simulink model "ASM_Traffic_V2X_Complete_Model_2"  (R2019a)
settings: Solver=ode1  StartTime=SIM.tstart.v  StopTime=Inf  FixedStep=SIM.StepSize.v  RelTol=1e-3
PostLoadFcn:
  | if any(exist('dsrtsu_mdlpostloadfcn', 'file') ~= 0), dsrtsu_mdlpostloadfcn('Execute', bdroot); end
  | try, asm_mdl_postloadfcn(bdroot, 'UpdateModel', 2200); catch, disp(lasterr); end,
undefined symbols (not defined in the file): _SensorPnts_1, _SensorPnts_13, _SensorPnts_17, _SensorPnts_21, _SensorPnts_25, _SensorPnts_29, _SensorPnts_33, _SensorPnts_37, _SensorPnts_41, _SensorPnts_45, _SensorPnts_49, _SensorPnts_5, _SensorPnts_53, _SensorPnts_57, _SensorPnts_9, _to_, CPT, G5A, ITS, MDL, rad, s_to_rpm, SIM
libraries: simulink x169, ASM_VehicleDynamics_lib x126, ASM_Traffic_lib x83, ASM_Utils_lib x49, mdbs x45, ASM_Environment_lib x17, dspindex x12, dsaV2xLibraryAux x10, dsmpblib x6, dsaV2xAsn1Library x4, dsaV2xLibrary x4, ASM_BrakeHydraulics_lib x4
(part 13 of 36)

== system ASM_Traffic_V2X_Complete_Model_2/MDL/SoftECU/Soft_ECU_Engine_Basic/StarterPermanentOn_Handling ==
  ASMSignalBus_ : Inport
  Sw_Starter[0Off|1On]_ : Inport  Port=2
  Bus Selector : BusSelector  OutputSignals=Sw_Starter_Mode[1Stim|2PermanentOn]
  BusAssignment : BusAssignment  AssignedSignals=Sw_Starter[0Off|1On]
  StarterPermanantOn : simulink/Logic and Bit Operations/Compare To Constant  relop===  const=2  OutDataTypeStr=boolean
  Sw_StarterOn : Constant
  Switch : Switch  Criteria=u2 ~= 0
  ASMSignalBus : Outport
  Sw_Starter[0Off|1On] : Outport  Port=2
  wires:
  BusAssignment/1 -> ASMSignalBus/1  "EngineOperation"
  Switch/1 -> BusAssignment/2, Sw_Starter[0Off|1On]/1
  Bus Selector/1 -> StarterPermanantOn/1  "<Sw_Starter_Mode[1Stim|2PermanentOn]>"
  Sw_StarterOn/1 -> Switch/1
  StarterPermanantOn/1 -> Switch/2
  ASMSignalBus_/1 -> BusAssignment/1
  [TAG_StartButton_Signals] -> Bus Selector/1
  Sw_Starter[0Off|1On]_/1 -> Switch/3

== system ASM_Traffic_V2X_Complete_Model_2/MDL/SoftECU/Soft_ECU_Engine_Basic/Torque_Intervention_During_Gear_Shift ==
  Factor_Trq_Engine_Red[%] : Inport
  Pos_AccPedal_Driver[%] : Inport  Port=2
  Product : Product
  Saturation[0_100] : Saturate  UpperLimit=100  LowerLimit=0
  UnitConversion : ASM_Utils_lib/UnitConversion/UnitConversion  Selection=%_to_[0_1]
  Pos_AccPedal[%] : Outport
  wires:
  Pos_AccPedal_Driver[%]/1 -> Product/2
  UnitConversion/1 -> Product/1
  Saturation[0_100]/1 -> Pos_AccPedal[%]/1
  Product/1 -> Saturation[0_100]/1
  Factor_Trq_Engine_Red[%]/1 -> UnitConversion/1

== system ASM_Traffic_V2X_Complete_Model_2/MDL/SoftECU/Soft_ECU_Transmission/ASMSignalCollector ==
  BusCreator : BusCreator  Inputs=5
  ASMSignalBus : Outport
  wires:
  BusCreator/1 -> ASMSignalBus/1  "SoftECU_Transmission"
  [ASMBUS_SOFTECU_LOCKUP_CLUTCH_CONTROL] -> BusCreator/1
  [ASMBUS_SOFTECU_SHIFT_LOCK_CONTROL] -> BusCreator/2
  [ASMBUS_SOFTECU_SHIFT_STRATEGY] -> BusCreator/3
  [ASMBUS_SOFTECU_TIP_SHIFT_CONTROL] -> BusCreator/4
  [ASMBUS_SOFTECU_TORQUE_INTERVENTION_CONTROL] -> BusCreator/5

== system ASM_Traffic_V2X_Complete_Model_2/MDL/SoftECU/Soft_ECU_Transmission/SOFTECU_SETUP ==
  Gear_Max_Maneuver[0Off|1_n] : Inport
  SOFTECU_TRANSMISSION_SETUP : ASM_VehicleDynamics_lib/SoftECU/SoftECU_Transmission/SOFTECU_TRANSMISSION_SETUP  Tag=ASM_SUBCOMPONENT  Const_Max_num_Gear=MDL.SoftECU.SoftECUTransmission.Const_Max_num_Gear  ASMProperties=struct('Name','SOFTECU_TRANSMISSION_SETUP','Version','1.0','Library','ASM_VehicleDynamics_lib')  ASMInstanceName=softecu_transmission_setup  ASMInstanceID=1
  Terminator : Terminator
  tag scope: TAG_SoftECU_Const_Max_num_Gear=global
  wires:
  SOFTECU_TRANSMISSION_SETUP/1 -> [TAG_SoftECU_Const_Max_num_Gear]
  [TAG_SoftECU_Const_Max_num_Gear] -> Terminator/1
  Gear_Max_Maneuver[0Off|1_n]/1 -> SOFTECU_TRANSMISSION_SETUP/1

== system ASM_Traffic_V2X_Complete_Model_2/MDL/SoftECU/Soft_ECU_Transmission/Sw_Gear ==
  In[] : Inport
  Ext : Constant
  OR : Logic  Operator=OR  AllPortsSameDT=off  OutDataTypeStr=boolean
  Ref : simulink/Logic and Bit Operations/Compare To Constant  relop===  const=4  OutDataTypeStr=boolean
  SoftECU : Constant  Value=2
  Stim : simulink/Logic and Bit Operations/Compare To Constant  relop===  const=1  OutDataTypeStr=boolean
  Switch : Switch  Criteria=u2 ~= 0
  Terminator : Terminator
  Sw_Gear[] : Outport
  wires:
  Switch/1 -> Terminator/1
  SoftECU/1 -> Switch/3, Sw_Gear[]/1
  Ext/1 -> Switch/1
  OR/1 -> Switch/2
  Ref/1 -> OR/2
  Stim/1 -> OR/1
  In[]/1 -> Ref/1, Stim/1

== system ASM_Traffic_V2X_Complete_Model_2/MDL/SoftECU/Soft_ECU_Transmission/Sw_LockupClutch ==
  In[] : Inport
  SoftECU : Constant  Value=2
  Terminator : Terminator
  Sw_LockupClutch[] : Outport
  wires:
  SoftECU/1 -> Sw_LockupClutch[]/1
  In[]/1 -> Terminator/1

== system ASM_Traffic_V2X_Complete_Model_2/MDL/VehicleDynamics/Brake/ASMSignalCollector ==
  BusCreator3 : BusCreator  Inputs=5
  ASMSignalBus : Outport
  wires:
  BusCreator3/1 -> ASMSignalBus/1  "Brake"
  [ASMBUS_VehicleDynamics_BrakeHydraulics] -> BusCreator3/2
  [TAG_DISP_BrkHyd_MasterBrakeCylinder] -> BusCreator3/1
  [ASMBUS_VehicleDynamics_BrakeDisc] -> BusCreator3/3
  [ASMBUS_VehicleDynamics_BrakeBooster] -> BusCreator3/4
  [ASMBUS_VehicleDynamics_Manifold] -> BusCreator3/5

== system ASM_Traffic_V2X_Complete_Model_2/MDL/VehicleDynamics/Brake/BRAKE_HYDRAULICS ==
  p_MasterBrakeCylinder[bar] : Inport
  Sw_DistributionPattern[1X|2II] : Inport  Port=2
  Reset[] : Inport  Port=3
  Ctrl_HydPump[0_1] : Inport  Port=4
  Ctrl_PreChargeValve_1[] : Inport  Port=5
  Ctrl_PreChargeValve_2[] : Inport  Port=6
  Ctrl_ChangeOverValve_1[] : Inport  Port=7
  Ctrl_ChangeOverValve_2[] : Inport  Port=8
  Ctrl_InletValve_FL[] : Inport  Port=9
  Ctrl_InletValve_FR[] : Inport  Port=10
  Ctrl_InletValve_RL[] : Inport  Port=11
  Ctrl_InletValve_RR[] : Inport  Port=12
  Ctrl_OutletValve_FL[] : Inport  Port=13
  Ctrl_OutletValve_FR[] : Inport  Port=14
  Ctrl_OutletValve_RL[] : Inport  Port=15
  Ctrl_OutletValve_RR[] : Inport  Port=16
  ECU_Mode[0None|1ABS|2ESP|3ASR] : Inport  Port=17
  p_Ambient[bar] : Inport  Port=18
  ASMSignalCollector : Subsystem
  BRAKING_CIRCUIT_BASIC : ASM_BrakeHydraulics_lib/BrakeHydraulics/BrakingCircuitBasic/BRAKING_CIRCUIT_BASIC  Tag=ASM_SUBCOMPONENT  Const_TimeConst=MDL.BrkHyd.BrakeHydraulicsBasic.Const_TimeConst  StepSize=SIM.StepSize  ASMProperties=struct('Name','BRAKING_CIRCUIT_BASIC','Version','4.0','Library','ASM_BrakeHydraulics_lib')  ASMInstanceName=braking_circuit_basic  ASMInstanceID=1
  Mux : Mux
  Mux1 : Mux
  Terminator_{1..2,4,8,11,14} (6 alike) : Terminator
  ASMSignalBus : Outport
  p_Brake[FL,FR,RL,RR][bar] : Outport  Port=2
  tag scope: TAG_DISP_BrkHyd_BrakingCircuitBasic=global
  wires:
  Sw_DistributionPattern[1X|2II]/1 -> Terminator_14/1
  BRAKING_CIRCUIT_BASIC/2 -> p_Brake[FL,FR,RL,RR][bar]/1
  BRAKING_CIRCUIT_BASIC/1 -> [TAG_DISP_BrkHyd_BrakingCircuitBasic]
  Reset[]/1 -> BRAKING_CIRCUIT_BASIC/2
  ASMSignalCollector/1(ASMSignalBus) -> ASMSignalBus/1
  Ctrl_HydPump[0_1]/1 -> Terminator_4/1
  Ctrl_PreChargeValve_1[]/1 -> Terminator_1/1
  Ctrl_ChangeOverValve_1[]/1 -> Terminator_2/1
  Ctrl_PreChargeValve_2[]/1 -> Terminator_11/1
  Ctrl_ChangeOverValve_2[]/1 -> Terminator_8/1
  ECU_Mode[0None|1ABS|2ESP|3ASR]/1 -> BRAKING_CIRCUIT_BASIC/4
  Ctrl_InletValve_FL[]/1 -> Mux/1
  Ctrl_InletValve_FR[]/1 -> Mux/2
  Ctrl_InletValve_RL[]/1 -> Mux/3
  Ctrl_InletValve_RR[]/1 -> Mux/4
  Ctrl_OutletValve_RR[]/1 -> Mux1/4
  Ctrl_OutletValve_RL[]/1 -> Mux1/3
  Ctrl_OutletValve_FR[]/1 -> Mux1/2
  Ctrl_OutletValve_FL[]/1 -> Mux1/1
  Mux/1 -> BRAKING_CIRCUIT_BASIC/5
  Mux1/1 -> BRAKING_CIRCUIT_BASIC/6
  p_Ambient[bar]/1 -> BRAKING_CIRCUIT_BASIC/3
  p_MasterBrakeCylinder[bar]/1 -> BRAKING_CIRCUIT_BASIC/1

== system ASM_Traffic_V2X_Complete_Model_2/MDL/VehicleDynamics/Brake/ForceParkingBrake ==
  Sw_ParkingBrake[0Off|1On] : Inport
  F_ParkingBrake_Off[FL;FR;RL;RR][N] : Constant  Value=[0, 0, 0, 0]
  F_ParkingBrake_On[FL;FR;RL;RR][N] : Constant  Value=[0, 0, 10000, 10000]
  Switch : Switch  Threshold=0.5
  F_ParkingBrake[FL;FR;RL;RR][N] : Outport
  wires:
  Switch/1 -> F_ParkingBrake[FL;FR;RL;RR][N]/1
  F_ParkingBrake_On[FL;FR;RL;RR][N]/1 -> Switch/1
  F_ParkingBrake_Off[FL;FR;RL;RR][N]/1 -> Switch/3
  Sw_ParkingBrake[0Off|1On]/1 -> Switch/2

== system ASM_Traffic_V2X_Complete_Model_2/MDL/VehicleDynamics/Brake/OpenBrkHydModel ==

== system ASM_Traffic_V2X_Complete_Model_2/MDL/VehicleDynamics/CommonVehicleParameters/Rename1 ==
  In1 : Inport
  Out1 : Outport
  wires:
  In1/1 -> Out1/1

== system ASM_Traffic_V2X_Complete_Model_2/MDL/VehicleDynamics/CommonVehicleParameters/Rename2 ==
  In1 : Inport
  Out1 : Outport
  wires:
  In1/1 -> Out1/1

== system ASM_Traffic_V2X_Complete_Model_2/MDL/VehicleDynamics/CommonVehicleParameters/Rename3 ==
  In1 : Inport
  Out1 : Outport
  wires:
  In1/1 -> Out1/1

== system ASM_Traffic_V2X_Complete_Model_2/MDL/VehicleDynamics/CommonVehicleParameters/Rename4 ==
  In1 : Inport
  Out1 : Outport
  wires:
  In1/1 -> Out1/1

== system ASM_Traffic_V2X_Complete_Model_2/MDL/VehicleDynamics/CommonVehicleParameters/Rename5 ==
  In1 : Inport
  Out1 : Outport
  wires:
  In1/1 -> Out1/1

== system ASM_Traffic_V2X_Complete_Model_2/MDL/VehicleDynamics/CommonVehicleParameters/Rename6 ==
  In1 : Inport
  Out1 : Outport
  wires:
  In1/1 -> Out1/1

== system ASM_Traffic_V2X_Complete_Model_2/MDL/VehicleDynamics/CommonVehicleParameters/Rename7 ==
  In1 : Inport
  Out1 : Outport
  wires:
  In1/1 -> Out1/1

== system ASM_Traffic_V2X_Complete_Model_2/MDL/VehicleDynamics/CommonVehicleParameters/Rename8 ==
  In1 : Inport
  Out1 : Outport
  wires:
  In1/1 -> Out1/1

== system ASM_Traffic_V2X_Complete_Model_2/MDL/VehicleDynamics/Suspension/ASMSignalCollector ==
  BusCreator1 : BusCreator  Inputs=2
  ASMSignalBus : Outport
  wires:
  [ASMBUS_SuspensionRear] -> BusCreator1/2
  [ASMBUS_SuspensionFront] -> BusCreator1/1
  BusCreator1/1 -> ASMSignalBus/1  "Suspension"

== system ASM_Traffic_V2X_Complete_Model_2/MDL/VehicleDynamics/Suspension/SuspensionFront ==
  q_Wheel_dt[q1_Front;q2_Front;q1_Rear;q2_Rear][] : Inport
  q_Wheel[q1_Front;q2_Front;q1_Rear;q2_Rear][] : Inport  Port=2
  F_Tire[FL;FR;RL;RR][x;y;z][N] : Inport  Port=3
  Trq_Tire[FL;FR;RL;RR][x;y;z][N|m] : Inport  Port=4
  AirSuspensionSignals_In : Inport  Port=5
  Reset[] : Inport  Port=6
  ASMSignalCollector : Subsystem
  Bus Creator1 : BusCreator  Inputs=8
  Bus Selector4 : BusSelector  OutputSignals=Displ_SteeringRod[Displ;Displ_dt][m;m|s]  OutputAsBus=on
  Constant : Constant  Value=0
  Constant1 : Constant  Value=[0;0]
  Constant2 : Constant  Value=0
  Demux : Demux  Outputs=[1 1]
  Demux1 : Demux  Outputs=[1 1]
  Demux2 : Demux  Outputs=2
  F_FL_dDispl_external[N|m] : Constant  Value=0
  F_FL_external[N] : Constant  Value=0
  F_FR_dDispl_external[N|m] : Constant  Value=0
  F_FR_external[N] : Constant  Value=0
  Mux : Mux  Inputs=2
  Mux1 : Mux  Inputs=2
  Mux2 : Mux  Inputs=2
  OpenSusKinFrontModel : Subsystem
      settings: OpenFcn=asm_open_lib('ASM_VehicleDynamics_lib/VehicleDynamics/Suspension/Front/SuspensionKinematics');
      mask Display: disp('Open\nASM_VehicleDynamics_lib\nSuspension Kinematics Front')
  RELATIVE_POSITION_FRONT : ASM_VehicleDynamics_lib/VehicleDynamics/Suspension/Front/CommonSuspensionBlocks/RELATIVE_POSITION_FRONT  Tag=ASM_SUBCOMPONENT  ASMProperties=struct('Name','RELATIVE_POSITION_FRONT','Version','6.0','Library','ASM_VehicleDynamics_lib')  ASMInstanceName=relative_position_front  ASMInstanceID=1
  RELATIVE_VELOCITIES_FRONT : ASM_VehicleDynamics_lib/VehicleDynamics/Suspension/Front/CommonSuspensionBlocks/RELATIVE_VELOCITIES_FRONT  Tag=ASM_SUBCOMPONENT  ASMProperties=struct('Name','RELATIVE_VELOCITIES_FRONT','Version','3.0','Library','ASM_VehicleDynamics_lib')  ASMInstanceName=relative_velocities_front  ASMInstanceID=1
  STABI_COMP_FRONT : ASM_VehicleDynamics_lib/VehicleDynamics/Suspension/Front/CommonSuspensionBlocks/STABI_COMP_FRONT  ASMProperties=struct('Name','STABI_COMP_FRONT','Version','1.0','Library','ASM_VehicleDynamics_lib')  ASMInstanceName=stabi_comp_front  ASMInstanceID=1
  SUSCOMP_2D_FRONT : ASM_VehicleDynamics_lib/VehicleDynamics/Suspension/Front/CommonSuspensionBlocks/SUSCOMP_2D_FRONT  Tag=ASM_SUBCOMPONENT  Map_Displ_x_Wheel_F_x=MDL.VehicleDynamics.SuspensionCompliance.Front.Map_Displ_x_Wheel_F_x_2d  Map_Displ_x_Wheel_F_y=MDL.VehicleDynamics.SuspensionCompliance.Front.Map_Displ_x_Wheel_F_y_2d  Map_Displ_x_Wheel_Trq_x=MDL.VehicleDynamics.SuspensionCompliance.Front.Map_Displ_x_Wheel_Trq_x_2d  Map_Displ_x_Wheel_Trq_y=MDL.VehicleDynamics.SuspensionCompliance.Front.Map_Displ_x_Wheel_Trq_y_2d  Map_Displ_x_Wheel_Trq_z=MDL.VehicleDynamics.SuspensionCompliance.Front.Map_Displ_x_Wheel_Trq_z_2d  Map_Displ_y_Wheel_F_x=MDL.VehicleDynamics.SuspensionCompliance.Front.Map_Displ_y_Wheel_F_x_2d  Map_Displ_y_Wheel_F_y=MDL.VehicleDynamics.SuspensionCompliance.Front.Map_Displ_y_Wheel_F_y_2d  Map_Displ_y_Wheel_Trq_x=MDL.VehicleDynamics.SuspensionCompliance.Front.Map_Displ_y_Wheel_Trq_x_2d  Map_Displ_y_Wheel_Trq_y=MDL.VehicleDynamics.SuspensionCompliance.Front.Map_Displ_y_Wheel_Trq_y_2d  Map_Displ_y_Wheel_Trq_z=MDL.VehicleDynamics.SuspensionCompliance.Front.Map_Displ_y_Wheel_Trq_z_2d  Map_Angle_Alpha_Wheel_F_x=MDL.VehicleDynamics.SuspensionCompliance.Front.Map_Angle_AlphaCamber_Wheel_F_x_2d  Map_Angle_Alpha_Wheel_F_y=MDL.VehicleDynamics.SuspensionCompliance.Front.Map_Angle_AlphaCamber_Wheel_F_y_2d  Map_Angle_Alpha_Wheel_Trq_x=MDL.VehicleDynamics.SuspensionCompliance.Front.Map_Angle_AlphaCamber_Wheel_Trq_x_2d  Map_Angle_Alpha_Wheel_Trq_y=MDL.VehicleDynamics.SuspensionCompliance.Front.Map_Angle_AlphaCamber_Wheel_Trq_y_2d  Map_Angle_Alpha_Wheel_Trq_z=MDL.VehicleDynamics.SuspensionCompliance.Front.Map_Angle_AlphaCamber_Wheel_Trq_z_2d  Map_Angle_Gamma_Wheel_F_x=MDL.VehicleDynamics.SuspensionCompliance.Front.Map_Angle_GammaToe_Wheel_F_x_2d  Map_Angle_Gamma_Wheel_F_y=MDL.VehicleDynamics.SuspensionCompliance.Front.Map_Angle_GammaToe_Wheel_F_y_2d  Map_Angle_Gamma_Wheel_Trq_x=MDL.VehicleDynamics.SuspensionCompliance.Front.Map_Angle_GammaToe_Wheel_Trq_x_2d  Map_Angle_Gamma_Wheel_Trq_y=MDL.VehicleDynamics.SuspensionCompliance.Front.Map_Angle_GammaToe_Wheel_Trq_y_2d  Map_Angle_Gamma_Wheel_Trq_z=MDL.VehicleDynamics.SuspensionCompliance.Front.Map_Angle_GammaToe_Wheel_Trq_z_2d  Const_NaturalFrequency_Displ_x=MDL.VehicleDynamics.SuspensionCompliance.Front.Const_NaturalFrequency_Displ_x  Const_NaturalFrequency_Displ_y=MDL.VehicleDynamics.SuspensionCompliance.Front.Const_NaturalFrequency_Displ_y  Const_NaturalFrequency_Angle_Alpha=MDL.VehicleDynamics.SuspensionCompliance.Front.Const_NaturalFrequency_Angle_AlphaCamber  Const_NaturalFrequency_Angle_Gamma=MDL.VehicleDynamics.SuspensionCompliance.Front.Const_NaturalFrequency_Angle_GammaToe  StepSize=SIM.StepSize  ASMProperties=struct('Name','SUSCOMP_2D_FRONT','Version','3.0','Library','ASM_VehicleDynamics_lib')  ASMInstanceName=suscomp_2d_front  ASMInstanceID=1
  SUSPENSION_FORCES_FRONT : ASM_VehicleDynamics_lib/VehicleDynamics/Suspension/Front/CommonSuspensionBlocks/SUSPENSION_FORCES_FRONT  Tag=ASM_SUBCOMPONENT  Map_Force_Left_Spring=MDL.VehicleDynamics.Suspension.Front.Map_Force_LeftSpring  Map_Force_Left_Damper=MDL.VehicleDynamics.Suspension.Front.Map_Force_LeftDamper  Map_Force_Right_Spring=MDL.VehicleDynamics.Suspension.Front.Map_Force_RightSpring  Map_Force_Right_Damper=MDL.VehicleDynamics.Suspension.Front.Map_Force_RightDamper  Map_Force_Stabilizer=MDL.VehicleDynamics.Suspension.Front.Map_Force_Stabilizer  ASMProperties=struct('Name','SUSPENSION_FORCES_FRONT','Version','4.0','Library','ASM_VehicleDynamics_lib')  ASMInstanceName=SusForcesFront  ASMInstanceID=1
  SUSPENSION_FORCE_KINEMATICS_FRONT : ASM_VehicleDynamics_lib/VehicleDynamics/Suspension/Front/CommonSuspensionBlocks/SUSPENSION_FORCE_KINEMATICS_FRONT  Tag=ASM_SUBCOMPONENT  StepSize=SIM.StepSize  ASMProperties=struct('Name','SUSPENSION_FORCE_KINEMATICS_FRONT','Version','4.0','Library','ASM_VehicleDynamics_lib')  ASMInstanceName=suspension_force_kinematics_front  ASMInstanceID=1
  SUSPENSION_KINEMATICS_FRONT_SYMMETRIC : ASM_VehicleDynamics_lib/VehicleDynamics/Suspension/Front/SuspensionKinematics/SUSPENSION_KINEMATICS_FRONT_SYMMETRIC  Tag=ASM_SUBCOMPONENT  Const_TrackWidth_Front=MDL.VehicleDynamics.Suspension.Front.TableBased.Const_TrackWidth_Front  Map_Displ_x_Wheel=MDL.VehicleDynamics.Suspension.Front.TableBased.Map_Displ_x_Wheel  Map_Displ_y_Wheel=MDL.VehicleDynamics.Suspension.Front.TableBased.Map_Displ_y_Wheel  Map_Angle_Alpha_Wheel=MDL.VehicleDynamics.Suspension.Front.TableBased.Map_Angle_AlphaCamber_Wheel  Map_Angle_Beta_Wheel=MDL.VehicleDynamics.Suspension.Front.TableBased.Map_Angle_BetaSideView_Wheel  Map_Angle_Gamma_Wheel=MDL.VehicleDynamics.Suspension.Front.TableBased.Map_Angle_GammaToe_Wheel  Map_Displ_Spring=MDL.VehicleDynamics.Suspension.Front.TableBased.Map_Displ_Spring  Map_Displ_Damper=MDL.VehicleDynamics.Suspension.Front.TableBased.Map_Displ_Damper  Map_Displ_Stabilizer=MDL.VehicleDynamics.Suspension.Front.TableBased.Map_Displ_Stabilizer  ASMProperties=struct('Name','SUSPENSION_KINEMATICS_FRONT_SYMMETRIC','Version','10.0','Library','ASM_VehicleDynamics_lib')  ASMInstanceName=SusKinFrontSym  ASMInstanceID=1
  Selector : Selector  InputPortWidth=4  IndexOptions=Index vector (dialog)  Indices=[1 2]  OutputSizes=1
  Selector1 : Selector  InputPortWidth=12  IndexOptions=Index vector (dialog)  Indices=[1 4]  OutputSizes=1
  Selector10 : Selector  InputPortWidth=12  IndexOptions=Index vector (dialog)  Indices=[1 4]  OutputSizes=1
  Selector2 : Selector  InputPortWidth=12  IndexOptions=Index vector (dialog)  Indices=[2 5]  OutputSizes=1
  Selector3 : Selector  InputPortWidth=12  IndexOptions=Index vector (dialog)  Indices=[3 6]  OutputSizes=1
  Selector4 : Selector  InputPortWidth=12  IndexOptions=Index vector (dialog)  Indices=[2 5]  OutputSizes=1
  Selector8 : Selector  InputPortWidth=4  IndexOptions=Index vector (dialog)  Indices=[1 2]  OutputSizes=1
  Sum{,1..3} (4 alike) : Sum  Inputs=++|
  Sum4 : Sum  Inputs=|++
  Terminator : Terminator
  zeros : Constant  Value=zeros(6,1)
  "Pos_Wheel[FL,FR][x;y;z][m] " : Outport
  UnitVec_y_Wheel_CoorSys_V[FL,FR][x;y;z] : Outport  Port=2
  v_Rel_WheelBody[FL,FR][x;y;z][m|s] : Outport  Port=3
  w_Rel_WheelBody[FL,FR][x;y;z][rad|s] : Outport  Port=4
  gF_Front_Susp[q1,q2][] : Outport  Port=5
  gFront_dq_Front_dt[2x2][] : Outport  Port=6
  SuspensionKinematicRelations_Front : Outport  Port=7
  AirSuspensionSignals_Front : Outport  Port=8
  tag scope: ASMBUS_SuspensionComplianceFront=global, ASMBUS_SuspensionForcesFront=global, ASMBUS_SuspensionForcesKinematicsFront=global, ASMBUS_SuspensionKinematicsFront=global, ASMBUS_WheelRelativePositionFront=global, ASMBUS_WheelRelativeVelocityFront=global
  wires:
  Selector4/1 -> SUSCOMP_2D_FRONT/4
  Bus Selector4/1 -> Demux2/1
  [TAG_FromIO_Steering] -> Bus Selector4/1
  STABI_COMP_FRONT/1 -> Sum4/2
  Sum4/1 -> SUSCOMP_2D_FRONT/5
  Selector3/1 -> Sum4/1
  SUSPENSION_KINEMATICS_FRONT_SYMMETRIC/22 -> STABI_COMP_FRONT/1
  Constant2/1 -> AirSuspensionSignals_Front/1
  AirSuspensionSignals_In/1 -> Terminator/1
  Sum3/1 -> SUSPENSION_FORCE_KINEMATICS_FRONT/8
  Sum2/1 -> SUSPENSION_FORCE_KINEMATICS_FRONT/7
  F_FR_dDispl_external[N|m]/1 -> Sum3/1
  F_FR_external[N]/1 -> Sum2/1
  F_FL_dDispl_external[N|m]/1 -> Sum1/1
  Sum1/1 -> SUSPENSION_FORCE_KINEMATICS_FRONT/2
  F_FL_external[N]/1 -> Sum/1
  Sum/1 -> SUSPENSION_FORCE_KINEMATICS_FRONT/1
  Selector10/1 -> SUSCOMP_2D_FRONT/3
  Selector2/1 -> SUSCOMP_2D_FRONT/2
  Selector1/1 -> SUSCOMP_2D_FRONT/1
  Selector8/1 -> Demux1/1
  Selector/1 -> Demux/1
  zeros/1 -> SUSCOMP_2D_FRONT/8
  [TAG_SW_Rotation] -> SUSCOMP_2D_FRONT/7, SUSPENSION_KINEMATICS_FRONT_SYMMETRIC/7, RELATIVE_POSITION_FRONT/9
  Demux2/2 -> Mux2/1, Mux2/2
  Demux2/1 -> Mux/1, Mux/2
  Constant1/1 -> SUSPENSION_FORCE_KINEMATICS_FRONT/21, SUSPENSION_FORCE_KINEMATICS_FRONT/20
  Trq_Tire[FL;FR;RL;RR][x;y;z][N|m]/1 -> Selector3/1, Selector4/1, Selector10/1
  Constant/1 -> SUSPENSION_FORCE_KINEMATICS_FRONT/19, SUSPENSION_FORCE_KINEMATICS_FRONT/18, SUSPENSION_FORCE_KINEMATICS_FRONT/17, SUSPENSION_FORCE_KINEMATICS_FRONT/16
  Reset[]/1 -> SUSCOMP_2D_FRONT/6
  SUSPENSION_FORCE_KINEMATICS_FRONT/2 -> Mux1/1
  SUSPENSION_KINEMATICS_FRONT_SYMMETRIC/1 -> [ASMBUS_SuspensionKinematicsFront]
  SUSPENSION_FORCE_KINEMATICS_FRONT/1 -> [ASMBUS_SuspensionForcesKinematicsFront]
  Demux1/1 -> SUSPENSION_KINEMATICS_FRONT_SYMMETRIC/3
  Demux1/2 -> SUSPENSION_KINEMATICS_FRONT_SYMMETRIC/4
  Demux/1 -> SUSPENSION_KINEMATICS_FRONT_SYMMETRIC/5, RELATIVE_VELOCITIES_FRONT/2
  Demux/2 -> SUSPENSION_KINEMATICS_FRONT_SYMMETRIC/6, RELATIVE_VELOCITIES_FRONT/3
  RELATIVE_VELOCITIES_FRONT/3 -> w_Rel_WheelBody[FL,FR][x;y;z][rad|s]/1
  RELATIVE_VELOCITIES_FRONT/2 -> v_Rel_WheelBody[FL,FR][x;y;z][m|s]/1
  RELATIVE_POSITION_FRONT/1 -> [ASMBUS_WheelRelativePositionFront]
  Bus Creator1/1 -> SuspensionKinematicRelations_Front/1  "SuspensionKinematicRelations_Front"
  SUSPENSION_KINEMATICS_FRONT_SYMMETRIC/9 -> Bus Creator1/8, STABI_COMP_FRONT/3, RELATIVE_VELOCITIES_FRONT/15  "w_Rel_FR_Wheel_dDispl_SteeringRod_dt[x;y;z][rad|m]"
  SUSPENSION_KINEMATICS_FRONT_SYMMETRIC/8 -> RELATIVE_VELOCITIES_FRONT/14, Bus Creator1/7  "w_Rel_FR_Wheel_dq_Front[q1;q2][x;y;z][]"
  SUSPENSION_KINEMATICS_FRONT_SYMMETRIC/7 -> RELATIVE_VELOCITIES_FRONT/13, Bus Creator1/6  "Pos_FR_Wheel_dDispl_SteeringRod[x;y;z][]"
  SUSPENSION_KINEMATICS_FRONT_SYMMETRIC/6 -> RELATIVE_VELOCITIES_FRONT/12, Bus Creator1/5  "Pos_FR_Wheel_dq_Front[q1;q2][x;y;z][]"
  SUSPENSION_KINEMATICS_FRONT_SYMMETRIC/5 -> RELATIVE_VELOCITIES_FRONT/11, Bus Creator1/4, STABI_COMP_FRONT/2  "w_Rel_FL_Wheel_dDispl_SteeringRod_dt[x;y;z][rad|m]"
  SUSPENSION_KINEMATICS_FRONT_SYMMETRIC/4 -> RELATIVE_VELOCITIES_FRONT/10, Bus Creator1/3  "w_Rel_FL_Wheel_dq_Front_dt[q1;q2][x;y;z][]"
  SUSPENSION_KINEMATICS_FRONT_SYMMETRIC/3 -> RELATIVE_VELOCITIES_FRONT/9, Bus Creator1/2  "Pos_FL_Wheel_dDispl_SteeringRod[x;y;z][]"
  SUSPENSION_KINEMATICS_FRONT_SYMMETRIC/2 -> RELATIVE_VELOCITIES_FRONT/8, Bus Creator1/1  "Pos_FL_Wheel_dq_Front[q1;q2][x;y;z][]"
  q_Wheel[q1_Front;q2_Front;q1_Rear;q2_Rear][]/1 -> Selector8/1
  q_Wheel_dt[q1_Front;q2_Front;q1_Rear;q2_Rear][]/1 -> Selector/1
  Mux/1 -> SUSPENSION_KINEMATICS_FRONT_SYMMETRIC/1
  SUSPENSION_FORCE_KINEMATICS_FRONT/4 -> gFront_dq_Front_dt[2x2][]/1
  Mux1/1 -> gF_Front_Susp[q1,q2][]/1
  SUSPENSION_FORCE_KINEMATICS_FRONT/3 -> Mux1/2
  RELATIVE_POSITION_FRONT/3 -> UnitVec_y_Wheel_CoorSys_V[FL,FR][x;y;z]/1
  RELATIVE_POSITION_FRONT/2 -> "Pos_Wheel[FL,FR][x;y;z][m] "/1
  SUSPENSION_KINEMATICS_FRONT_SYMMETRIC/21 -> SUSPENSION_FORCE_KINEMATICS_FRONT/15
  SUSPENSION_KINEMATICS_FRONT_SYMMETRIC/20 -> SUSPENSION_FORCE_KINEMATICS_FRONT/14
  SUSPENSION_KINEMATICS_FRONT_SYMMETRIC/19 -> SUSPENSION_FORCE_KINEMATICS_FRONT/13
  SUSPENSION_KINEMATICS_FRONT_SYMMETRIC/18 -> SUSPENSION_FORCE_KINEMATICS_FRONT/12
  SUSPENSION_KINEMATICS_FRONT_SYMMETRIC/17 -> SUSPENSION_FORCE_KINEMATICS_FRONT/11
  SUSPENSION_FORCES_FRONT/11 -> SUSPENSION_FORCE_KINEMATICS_FRONT/10
  SUSPENSION_FORCES_FRONT/10 -> SUSPENSION_FORCE_KINEMATICS_FRONT/9
  SUSPENSION_FORCES_FRONT/9 -> Sum3/2
  SUSPENSION_FORCES_FRONT/8 -> Sum2/2
  SUSPENSION_FORCES_FRONT/7 -> SUSPENSION_FORCE_KINEMATICS_FRONT/6
  SUSPENSION_FORCES_FRONT/6 -> SUSPENSION_FORCE_KINEMATICS_FRONT/5, STABI_COMP_FRONT/4
  SUSPENSION_FORCES_FRONT/5 -> SUSPENSION_FORCE_KINEMATICS_FRONT/4
  SUSPENSION_FORCES_FRONT/4 -> SUSPENSION_FORCE_KINEMATICS_FRONT/3
  SUSPENSION_FORCES_FRONT/3 -> Sum1/2
  SUSPENSION_FORCES_FRONT/2 -> Sum/2
  SUSPENSION_KINEMATICS_FRONT_SYMMETRIC/16 -> SUSPENSION_FORCES_FRONT/3
  SUSPENSION_KINEMATICS_FRONT_SYMMETRIC/15 -> SUSPENSION_FORCES_FRONT/2
  SUSPENSION_KINEMATICS_FRONT_SYMMETRIC/14 -> SUSPENSION_FORCES_FRONT/1
  SUSPENSION_KINEMATICS_FRONT_SYMMETRIC/13 -> RELATIVE_POSITION_FRONT/8
  SUSPENSION_KINEMATICS_FRONT_SYMMETRIC/12 -> RELATIVE_POSITION_FRONT/7
  SUSPENSION_KINEMATICS_FRONT_SYMMETRIC/11 -> RELATIVE_POSITION_FRONT/6
  SUSPENSION_KINEMATICS_FRONT_SYMMETRIC/10 -> RELATIVE_POSITION_FRONT/5
  SUSCOMP_2D_FRONT/9 -> RELATIVE_POSITION_FRONT/4
  SUSCOMP_2D_FRONT/8 -> RELATIVE_POSITION_FRONT/3
  SUSCOMP_2D_FRONT/7 -> RELATIVE_POSITION_FRONT/2
  SUSCOMP_2D_FRONT/6 -> RELATIVE_POSITION_FRONT/1
  SUSCOMP_2D_FRONT/5 -> RELATIVE_VELOCITIES_FRONT/7
  SUSCOMP_2D_FRONT/4 -> RELATIVE_VELOCITIES_FRONT/6
  SUSCOMP_2D_FRONT/3 -> RELATIVE_VELOCITIES_FRONT/5
  SUSCOMP_2D_FRONT/2 -> RELATIVE_VELOCITIES_FRONT/4
  RELATIVE_VELOCITIES_FRONT/1 -> [ASMBUS_WheelRelativeVelocityFront]
  F_Tire[FL;FR;RL;RR][x;y;z][N]/1 -> Selector2/1, Selector1/1
  Mux2/1 -> SUSPENSION_KINEMATICS_FRONT_SYMMETRIC/2, RELATIVE_VELOCITIES_FRONT/1
  SUSCOMP_2D_FRONT/1 -> [ASMBUS_SuspensionComplianceFront]
  SUSPENSION_FORCES_FRONT/1 -> [ASMBUS_SuspensionForcesFront]

== system ASM_Traffic_V2X_Complete_Model_2/MDL/VehicleDynamics/Suspension/SuspensionRear ==
  q_Wheel_dt[q1_Front;q2_Front;q1_Rear;q2_Rear][] : Inport
  q_Wheel[q1_Front;q2_Front;q1_Rear;q2_Rear][] : Inport  Port=2
  F_Tire[FL;FR;RL;RR][x;y;z][N] : Inport  Port=3
  Trq_Tire[FL;FR;RL;RR][x;y;z][N|m] : Inport  Port=4
  AirSuspensionSignals_In : Inport  Port=5
  Reset[] : Inport  Port=6
  ASMSignalCollector : Subsystem
  Bus Creator : BusCreator  Inputs=8
  Constant : Constant  Value=[0 0]
  Constant1 : Constant  Value=0
  Constant2 : Constant  Value=0
  Constant3 : Constant  Value=[0;0]
  Demux : Demux  Outputs=[1 1]
  Demux1 : Demux  Outputs=[1 1]
  F_RL_dDispl_external[N|m] : Constant  Value=0
  F_RL_external[N] : Constant  Value=0
  F_RR_dDispl_external[N|m] : Constant  Value=0
  F_RR_external[N] : Constant  Value=0
  Mux1 : Mux  Inputs=2
  OpenSusKinRearModel : Subsystem
      settings: OpenFcn=asm_open_lib('ASM_VehicleDynamics_lib/VehicleDynamics/Suspension/Rear/SuspensionKinematics');
      mask Display: disp('Open\nASM_VehicleDynamics_lib\nSuspension Kinematics Rear')
  RELATIVE_POSITION_REAR : ASM_VehicleDynamics_lib/VehicleDynamics/Suspension/Rear/CommonSuspensionBlocks/RELATIVE_POSITION_REAR  Tag=ASM_SUBCOMPONENT  ASMProperties=struct('Name','RELATIVE_POSITION_REAR','Version','6.0','Library','ASM_VehicleDynamics_lib')  ASMInstanceName=relative_position_rear  ASMInstanceID=1
  RELATIVE_VELOCITIES_REAR : ASM_VehicleDynamics_lib/VehicleDynamics/Suspension/Rear/CommonSuspensionBlocks/RELATIVE_VELOCITIES_REAR  Tag=ASM_SUBCOMPONENT  ASMProperties=struct('Name','RELATIVE_VELOCITIES_REAR','Version','3.0','Library','ASM_VehicleDynamics_lib')  ASMInstanceName=relative_velocities_rear  ASMInstanceID=1
  SUSCOMP_2D_REAR : ASM_VehicleDynamics_lib/VehicleDynamics/Suspension/Rear/CommonSuspensionBlocks/SUSCOMP_2D_REAR  Tag=ASM_SUBCOMPONENT  Map_Displ_x_Wheel_F_x=MDL.VehicleDynamics.SuspensionCompliance.Rear.Map_Displ_x_Wheel_F_x_2d  Map_Displ_x_Wheel_F_y=MDL.VehicleDynamics.SuspensionCompliance.Rear.Map_Displ_x_Wheel_F_y_2d  Map_Displ_x_Wheel_Trq_x=MDL.VehicleDynamics.SuspensionCompliance.Rear.Map_Displ_x_Wheel_Trq_x_2d  Map_Displ_x_Wheel_Trq_y=MDL.VehicleDynamics.SuspensionCompliance.Rear.Map_Displ_x_Wheel_Trq_y_2d  Map_Displ_x_Wheel_Trq_z=MDL.VehicleDynamics.SuspensionCompliance.Rear.Map_Displ_x_Wheel_Trq_z_2d  Map_Displ_y_Wheel_F_x=MDL.VehicleDynamics.SuspensionCompliance.Rear.Map_Displ_y_Wheel_F_x_2d  Map_Displ_y_Wheel_F_y=MDL.VehicleDynamics.SuspensionCompliance.Rear.Map_Displ_y_Wheel_F_y_2d  Map_Displ_y_Wheel_Trq_x=MDL.VehicleDynamics.SuspensionCompliance.Rear.Map_Displ_y_Wheel_Trq_x_2d  Map_Displ_y_Wheel_Trq_y=MDL.VehicleDynamics.SuspensionCompliance.Rear.Map_Displ_y_Wheel_Trq_y_2d  Map_Displ_y_Wheel_Trq_z=MDL.VehicleDynamics.SuspensionCompliance.Rear.Map_Displ_y_Wheel_Trq_z_2d  Map_Angle_Alpha_Wheel_F_x=MDL.VehicleDynamics.SuspensionCompliance.Rear.Map_Angle_AlphaCamber_Wheel_F_x_2d  Map_Angle_Alpha_Wheel_F_y=MDL.VehicleDynamics.SuspensionCompliance.Rear.Map_Angle_AlphaCamber_Wheel_F_y_2d  Map_Angle_Alpha_Wheel_Trq_x=MDL.VehicleDynamics.SuspensionCompliance.Rear.Map_Angle_AlphaCamber_Wheel_Trq_x_2d  Map_Angle_Alpha_Wheel_Trq_y=MDL.VehicleDynamics.SuspensionCompliance.Rear.Map_Angle_AlphaCamber_Wheel_Trq_y_2d  Map_Angle_Alpha_Wheel_Trq_z=MDL.VehicleDynamics.SuspensionCompliance.Rear.Map_Angle_AlphaCamber_Wheel_Trq_z_2d  Map_Angle_Gamma_Wheel_F_x=MDL.VehicleDynamics.SuspensionCompliance.Rear.Map_Angle_GammaToe_Wheel_F_x_2d  Map_Angle_Gamma_Wheel_F_y=MDL.VehicleDynamics.SuspensionCompliance.Rear.Map_Angle_GammaToe_Wheel_F_y_2d  Map_Angle_Gamma_Wheel_Trq_x=MDL.VehicleDynamics.SuspensionCompliance.Rear.Map_Angle_GammaToe_Wheel_Trq_x_2d  Map_Angle_Gamma_Wheel_Trq_y=MDL.VehicleDynamics.SuspensionCompliance.Rear.Map_Angle_GammaToe_Wheel_Trq_y_2d  Map_Angle_Gamma_Wheel_Trq_z=MDL.VehicleDynamics.SuspensionCompliance.Rear.Map_Angle_GammaToe_Wheel_Trq_z_2d  Const_NaturalFrequency_Displ_x=MDL.VehicleDynamics.SuspensionCompliance.Rear.Const_NaturalFrequency_Displ_x  Const_NaturalFrequency_Displ_y=MDL.VehicleDynamics.SuspensionCompliance.Rear.Const_NaturalFrequency_Displ_y  Const_NaturalFrequency_Angle_Alpha=MDL.VehicleDynamics.SuspensionCompliance.Rear.Const_NaturalFrequency_Angle_AlphaCamber  Const_NaturalFrequency_Angle_Gamma=MDL.VehicleDynamics.SuspensionCompliance.Rear.Const_NaturalFrequency_Angle_GammaToe  StepSize=SIM.StepSize  ASMProperties=struct('Name','SUSCOMP_2D_REAR','Version','3.0','Library','ASM_VehicleDynamics_lib')  ASMInstanceName=suscomp_2d_rear  ASMInstanceID=1
  SUSPENSION_FORCES_REAR : ASM_VehicleDynamics_lib/VehicleDynamics/Suspension/Rear/CommonSuspensionBlocks/SUSPENSION_FORCES_REAR  Tag=ASM_SUBCOMPONENT  Map_Force_Left_Spring=MDL.VehicleDynamics.Suspension.Rear.Map_Force_LeftSpring  Map_Force_Left_Damper=MDL.VehicleDynamics.Suspension.Rear.Map_Force_LeftDamper  Map_Force_Right_Spring=MDL.VehicleDynamics.Suspension.Rear.Map_Force_RightSpring  Map_Force_Right_Damper=MDL.VehicleDynamics.Suspension.Rear.Map_Force_RightDamper  Map_Force_Stabilizer=MDL.VehicleDynamics.Suspension.Rear.Map_Force_Stabilizer  ASMProperties=struct('Name','SUSPENSION_FORCES_REAR','Version','4.0','Library','ASM_VehicleDynamics_lib')  ASMInstanceName=SusForcesRear  ASMInstanceID=1
  SUSPENSION_FORCE_KINEMATICS_REAR : ASM_VehicleDynamics_lib/VehicleDynamics/Suspension/Rear/CommonSuspensionBlocks/SUSPENSION_FORCE_KINEMATICS_REAR  Tag=ASM_SUBCOMPONENT  StepSize=SIM.StepSize  ASMProperties=struct('Name','SUSPENSION_FORCE_KINEMATICS_REAR','Version','4.0','Library','ASM_VehicleDynamics_lib')  ASMInstanceName=suspension_force_kinematics_rear  ASMInstanceID=1
  SUSPENSION_KINEMATICS_REAR_SYMMETRIC : ASM_VehicleDynamics_lib/VehicleDynamics/Suspension/Rear/SuspensionKinematics/SUSPENSION_KINEMATICS_REAR_SYMMETRIC  Tag=ASM_SUBCOMPONENT  Const_WheelBase=MDL.VehicleDynamics.Suspension.Rear.TableBased.Const_WheelBase  Const_TrackWidth_Rear=MDL.VehicleDynamics.Suspension.Rear.TableBased.Const_TrackWidth_Rear  Const_Pos_z0_Rear=MDL.VehicleDynamics.Suspension.Rear.TableBased.Const_Pos_z0_Rear  Map_Displ_x_Wheel=MDL.VehicleDynamics.Suspension.Rear.TableBased.Map_Displ_x_Wheel  Map_Displ_y_Wheel=MDL.VehicleDynamics.Suspension.Rear.TableBased.Map_Displ_y_Wheel  Map_Angle_Alpha_Wheel=MDL.VehicleDynamics.Suspension.Rear.TableBased.Map_Angle_AlphaCamber_Wheel  Map_Angle_Beta_Wheel=MDL.VehicleDynamics.Suspension.Rear.TableBased.Map_Angle_BetaSideView_Wheel  Map_Angle_Gamma_Wheel=MDL.VehicleDynamics.Suspension.Rear.TableBased.Map_Angle_GammaToe_Wheel  Map_Displ_Spring=MDL.VehicleDynamics.Suspension.Rear.TableBased.Map_Displ_Spring  Map_Displ_Damper=MDL.VehicleDynamics.Suspension.Rear.TableBased.Map_Displ_Damper  Map_Displ_Stabilizer=MDL.VehicleDynamics.Suspension.Rear.TableBased.Map_Displ_Stabilizer  ASMProperties=struct('Name','SUSPENSION_KINEMATICS_REAR_SYMMETRIC','Version','10.0','Library','ASM_VehicleDynamics_lib')  ASMInstanceName=SusKinRearSym  ASMInstanceID=1
  Selector1 : Selector  InputPortWidth=12  IndexOptions=Index vector (dialog)  Indices=[8 11]  OutputSizes=1
  Selector11 : Selector  InputPortWidth=12  IndexOptions=Index vector (dialog)  Indices=[7 10]  OutputSizes=1
  Selector4 : Selector  InputPortWidth=4  IndexOptions=Index vector (dialog)  Indices=[3 4]  OutputSizes=1
  Selector5 : Selector  InputPortWidth=12  IndexOptions=Index vector (dialog)  Indices=[7 10]  OutputSizes=1
  Selector6 : Selector  InputPortWidth=12  IndexOptions=Index vector (dialog)  Indices=[8 11]  OutputSizes=1
  Selector7 : Selector  InputPortWidth=12  IndexOptions=Index vector (dialog)  Indices=[9 12]  OutputSizes=1
  Selector9 : Selector  InputPortWidth=4  IndexOptions=Index vector (dialog)  Indices=[3 4]  OutputSizes=1
  Sum{,1..3} (4 alike) : Sum  Inputs=++|
  Terminator : Terminator
  WheelPos_Offset[x;y;z][m] : Constant  Value=[0 0 0]
  zeros : Constant  Value=zeros(6,1)
  "Pos_Wheel[RL;RR][x;y;z][m] " : Outport
  UnitVec_y_Wheel_CoorSys_V[RL;RR][x;y;z][] : Outport  Port=2
  v_Rel_WheelBody[RL;RR][x;y;z][m|s] : Outport  Port=3
  w_Rel_WheelBody[RL,RR][x;y;z][rad|s] : Outport  Port=4
  gF_Rear_Susp[q1,q2][] : Outport  Port=5
  gRear_dq_Rear_dt[2x2][] : Outport  Port=6
  SuspensionKinematicRelations_Rear : Outport  Port=7
  AirSuspensionSignals_Rear : Outport  Port=8
  tag scope: ASMBUS_SuspensionComplianceRear=global, ASMBUS_SuspensionForceKinematicsRear=global, ASMBUS_SuspensionForcesRear=global, ASMBUS_SuspensionKinematicsRear=global, ASMBUS_SuspensionRelativePositionRear=global, ASMBUS_SuspensionRelativeVelocitiesRear=global
  wires:
  Selector1/1 -> SUSCOMP_2D_REAR/4
  Constant1/1 -> AirSuspensionSignals_Rear/1
  AirSuspensionSignals_In/1 -> Terminator/1
  Sum3/1 -> SUSPENSION_FORCE_KINEMATICS_REAR/8
  Sum2/1 -> SUSPENSION_FORCE_KINEMATICS_REAR/7
  F_RR_dDispl_external[N|m]/1 -> Sum3/1
  F_RR_external[N]/1 -> Sum2/1
  F_RL_dDispl_external[N|m]/1 -> Sum1/1
  Sum1/1 -> SUSPENSION_FORCE_KINEMATICS_REAR/2
  F_RL_external[N]/1 -> Sum/1
  Sum/1 -> SUSPENSION_FORCE_KINEMATICS_REAR/1
  SUSPENSION_FORCES_REAR/9 -> Sum3/2
  SUSPENSION_FORCES_REAR/8 -> Sum2/2
  SUSPENSION_FORCES_REAR/3 -> Sum1/2
  SUSPENSION_FORCES_REAR/2 -> Sum/2
  Selector7/1 -> SUSCOMP_2D_REAR/5
  Selector11/1 -> SUSCOMP_2D_REAR/3
  Selector6/1 -> SUSCOMP_2D_REAR/2
  Selector5/1 -> SUSCOMP_2D_REAR/1
  Selector4/1 -> Demux1/1
  Selector9/1 -> Demux/1
  zeros/1 -> SUSCOMP_2D_REAR/8
  [TAG_SW_Rotation] -> RELATIVE_POSITION_REAR/9, SUSPENSION_KINEMATICS_REAR_SYMMETRIC/8, SUSCOMP_2D_REAR/7
  Constant3/1 -> SUSPENSION_FORCE_KINEMATICS_REAR/21, SUSPENSION_FORCE_KINEMATICS_REAR/20
  Constant2/1 -> SUSPENSION_FORCE_KINEMATICS_REAR/16, SUSPENSION_FORCE_KINEMATICS_REAR/17, SUSPENSION_FORCE_KINEMATICS_REAR/19, SUSPENSION_FORCE_KINEMATICS_REAR/18
  Trq_Tire[FL;FR;RL;RR][x;y;z][N|m]/1 -> Selector1/1, Selector7/1, Selector11/1
  Reset[]/1 -> SUSCOMP_2D_REAR/6
  Demux1/1 -> SUSPENSION_KINEMATICS_REAR_SYMMETRIC/3
  Demux1/2 -> SUSPENSION_KINEMATICS_REAR_SYMMETRIC/4
  WheelPos_Offset[x;y;z][m]/1 -> SUSPENSION_KINEMATICS_REAR_SYMMETRIC/7
  SUSPENSION_KINEMATICS_REAR_SYMMETRIC/1 -> [ASMBUS_SuspensionKinematicsRear]
  Demux/2 -> SUSPENSION_KINEMATICS_REAR_SYMMETRIC/6, RELATIVE_VELOCITIES_REAR/3
  Demux/1 -> SUSPENSION_KINEMATICS_REAR_SYMMETRIC/5, RELATIVE_VELOCITIES_REAR/2
  RELATIVE_POSITION_REAR/1 -> [ASMBUS_SuspensionRelativePositionRear]
  RELATIVE_VELOCITIES_REAR/3 -> w_Rel_WheelBody[RL,RR][x;y;z][rad|s]/1
  RELATIVE_VELOCITIES_REAR/2 -> v_Rel_WheelBody[RL;RR][x;y;z][m|s]/1
  RELATIVE_POSITION_REAR/3 -> UnitVec_y_Wheel_CoorSys_V[RL;RR][x;y;z][]/1
  RELATIVE_POSITION_REAR/2 -> "Pos_Wheel[RL;RR][x;y;z][m] "/1
  SUSPENSION_FORCE_KINEMATICS_REAR/1 -> [ASMBUS_SuspensionForceKinematicsRear]
  SUSPENSION_FORCES_REAR/1 -> [ASMBUS_SuspensionForcesRear]
  F_Tire[FL;FR;RL;RR][x;y;z][N]/1 -> Selector6/1, Selector5/1
  Bus Creator/1 -> SuspensionKinematicRelations_Rear/1  "SuspensionKinematicRelations_Rear"
  SUSPENSION_KINEMATICS_REAR_SYMMETRIC/9 -> RELATIVE_VELOCITIES_REAR/15, Bus Creator/8  "w_Rel_RR_Wheel_dDispl_SteeringRod_dt[x;y;z][rad|m]"
  SUSPENSION_KINEMATICS_REAR_SYMMETRIC/8 -> RELATIVE_VELOCITIES_REAR/14, Bus Creator/7  "w_Rel_RR_Wheel_dq_Rear[q1;q2][x;y;z][]"
  SUSPENSION_KINEMATICS_REAR_SYMMETRIC/7 -> RELATIVE_VELOCITIES_REAR/13, Bus Creator/6  "Pos_RR_Wheel_dDispl_SteeringRod[x;y;z][]"
  SUSPENSION_KINEMATICS_REAR_SYMMETRIC/6 -> RELATIVE_VELOCITIES_REAR/12, Bus Creator/5  "Pos_RR_Wheel_dq_Rear[q1;q2][x;y;z][]"
  SUSPENSION_KINEMATICS_REAR_SYMMETRIC/5 -> RELATIVE_VELOCITIES_REAR/11, Bus Creator/4  "w_Rel_RL_Wheel_dDispl_SteeringRod_dt[x;y;z][rad|m]"
  SUSPENSION_KINEMATICS_REAR_SYMMETRIC/4 -> RELATIVE_VELOCITIES_REAR/10, Bus Creator/3  "w_Rel_RL_Wheel_dq_Rear_dt[q1;q2][x;y;z][]"
  SUSPENSION_KINEMATICS_REAR_SYMMETRIC/3 -> RELATIVE_VELOCITIES_REAR/9, Bus Creator/2  "Pos_RL_Wheel_dDispl_SteeringRod[x;y;z][]"
  SUSPENSION_KINEMATICS_REAR_SYMMETRIC/2 -> RELATIVE_VELOCITIES_REAR/8, Bus Creator/1  "Pos_RL_Wheel_dq_Rear[q1;q2][x;y;z][]"
  q_Wheel[q1_Front;q2_Front;q1_Rear;q2_Rear][]/1 -> Selector4/1
  q_Wheel_dt[q1_Front;q2_Front;q1_Rear;q2_Rear][]/1 -> Selector9/1
  SUSPENSION_FORCE_KINEMATICS_REAR/4 -> gRear_dq_Rear_dt[2x2][]/1
  Mux1/1 -> gF_Rear_Susp[q1,q2][]/1
  SUSPENSION_FORCE_KINEMATICS_REAR/3 -> Mux1/2
  SUSPENSION_FORCE_KINEMATICS_REAR/2 -> Mux1/1
  SUSPENSION_KINEMATICS_REAR_SYMMETRIC/21 -> SUSPENSION_FORCE_KINEMATICS_REAR/15
  SUSPENSION_KINEMATICS_REAR_SYMMETRIC/20 -> SUSPENSION_FORCE_KINEMATICS_REAR/14
  SUSPENSION_KINEMATICS_REAR_SYMMETRIC/19 -> SUSPENSION_FORCE_KINEMATICS_REAR/13
  SUSPENSION_KINEMATICS_REAR_SYMMETRIC/18 -> SUSPENSION_FORCE_KINEMATICS_REAR/12
  SUSPENSION_KINEMATICS_REAR_SYMMETRIC/17 -> SUSPENSION_FORCE_KINEMATICS_REAR/11
  SUSPENSION_FORCES_REAR/11 -> SUSPENSION_FORCE_KINEMATICS_REAR/10
  SUSPENSION_FORCES_REAR/10 -> SUSPENSION_FORCE_KINEMATICS_REAR/9
  SUSPENSION_FORCES_REAR/7 -> SUSPENSION_FORCE_KINEMATICS_REAR/6
  SUSPENSION_FORCES_REAR/6 -> SUSPENSION_FORCE_KINEMATICS_REAR/5
  SUSPENSION_FORCES_REAR/5 -> SUSPENSION_FORCE_KINEMATICS_REAR/4
  SUSPENSION_FORCES_REAR/4 -> SUSPENSION_FORCE_KINEMATICS_REAR/3
  SUSPENSION_KINEMATICS_REAR_SYMMETRIC/16 -> SUSPENSION_FORCES_REAR/3
  SUSPENSION_KINEMATICS_REAR_SYMMETRIC/15 -> SUSPENSION_FORCES_REAR/2
  SUSPENSION_KINEMATICS_REAR_SYMMETRIC/14 -> SUSPENSION_FORCES_REAR/1
  SUSPENSION_KINEMATICS_REAR_SYMMETRIC/13 -> RELATIVE_POSITION_REAR/8
  SUSPENSION_KINEMATICS_REAR_SYMMETRIC/12 -> RELATIVE_POSITION_REAR/7
  SUSPENSION_KINEMATICS_REAR_SYMMETRIC/11 -> RELATIVE_POSITION_REAR/6
  SUSPENSION_KINEMATICS_REAR_SYMMETRIC/10 -> RELATIVE_POSITION_REAR/5
  SUSCOMP_2D_REAR/9 -> RELATIVE_POSITION_REAR/4
  SUSCOMP_2D_REAR/8 -> RELATIVE_POSITION_REAR/3
  SUSCOMP_2D_REAR/7 -> RELATIVE_POSITION_REAR/2
  SUSCOMP_2D_REAR/6 -> RELATIVE_POSITION_REAR/1
  SUSCOMP_2D_REAR/5 -> RELATIVE_VELOCITIES_REAR/7
  SUSCOMP_2D_REAR/4 -> RELATIVE_VELOCITIES_REAR/6
  SUSCOMP_2D_REAR/3 -> RELATIVE_VELOCITIES_REAR/5
  SUSCOMP_2D_REAR/2 -> RELATIVE_VELOCITIES_REAR/4
  RELATIVE_VELOCITIES_REAR/1 -> [ASMBUS_SuspensionRelativeVelocitiesRear]
  Constant/1 -> SUSPENSION_KINEMATICS_REAR_SYMMETRIC/2, SUSPENSION_KINEMATICS_REAR_SYMMETRIC/1, RELATIVE_VELOCITIES_REAR/1
  SUSCOMP_2D_REAR/1 -> [ASMBUS_SuspensionComplianceRear]

== system ASM_Traffic_V2X_Complete_Model_2/MDL/VehicleDynamics/Tire/ASMSignalCollector ==
  Sw_Tire_Model : Inport
  ActiveTire_FL : Subsystem
  ActiveTire_FR : Subsystem
  ActiveTire_RL : Subsystem
  ActiveTire_RR : Subsystem
  Bus Selector : BusSelector  OutputSignals=r_FL_Tire[m],Pos_CP_FL_CoorSys_E[x;y][m]  OutputAsBus=on
  Bus Selector1 : BusSelector  OutputSignals=r_FR_Tire[m],Pos_CP_FR_CoorSys_E[x;y][m]  OutputAsBus=on
  Bus Selector2 : BusSelector  OutputSignals=r_RL_Tire[m],Pos_CP_RL_CoorSys_E[x;y][m]  OutputAsBus=on
  Bus Selector3 : BusSelector  OutputSignals=r_RR_Tire[m],Pos_CP_RR_CoorSys_E[x;y][m]  OutputAsBus=on
  BusCreator{1..2,4..5} (4 alike) : BusCreator  Inputs=3
  BusCreator3 : BusCreator  Inputs=5
  BusCreator6 : BusCreator  Inputs=1
  ASMSignalBus : Outport
  wires:
  [ASMBUS_VehicleDynamics_ContactPoint_RR_Tire] -> Bus Selector3/1
  Bus Selector3/1 -> BusCreator5/1  "ContactPoint"
  [ASMBUS_VehicleDynamics_ContactPoint_RL_Tire] -> Bus Selector2/1
  Bus Selector2/1 -> BusCreator4/1  "ContactPoint"
  [ASMBUS_VehicleDynamics_ContactPoint_FR_Tire] -> Bus Selector1/1
  Bus Selector1/1 -> BusCreator2/1  "ContactPoint"
  Bus Selector/1 -> BusCreator1/1  "ContactPoint"
  [ASMBUS_VehicleDynamics_ContactPoint_FL_Tire] -> Bus Selector/1
  ActiveTire_RL/1(ASMSignalBus) -> BusCreator4/3
  ActiveTire_RR/1(ASMSignalBus) -> BusCreator5/3
  [ASMBUS_VehicleDynamics_MF_RR_Tire] -> ActiveTire_RR/3(MagicFormular)
  [ASMBUS_VehicleDynamics_TMEasy_RR_Tire] -> ActiveTire_RR/2(TMEasy)
  [ASMBUS_VehicleDynamics_ForcesAndTorques_RR_Tire] -> BusCreator5/2
  [ASMBUS_VehicleDynamics_TMEasy_RL_Tire] -> ActiveTire_RL/2(TMEasy)
  [ASMBUS_VehicleDynamics_MF_RL_Tire] -> ActiveTire_RL/3(MagicFormular)
  [ASMBUS_VehicleDynamics_ForcesAndTorques_RL_Tire] -> BusCreator4/2
  ActiveTire_FR/1(ASMSignalBus) -> BusCreator2/3
  [ASMBUS_VehicleDynamics_MF_FR_Tire] -> ActiveTire_FR/3(MagicFormular)
  [ASMBUS_VehicleDynamics_TMEasy_FR_Tire] -> ActiveTire_FR/2(TMEasy)
  [ASMBUS_VehicleDynamics_ForcesAndTorques_FR_Tire] -> BusCreator2/2
  ActiveTire_FL/1(ASMSignalBus) -> BusCreator1/3
  [ASMBUS_VehicleDynamics_MF_FL_Tire] -> ActiveTire_FL/3(MagicFormular)
  [ASMBUS_VehicleDynamics_TMEasy_FL_Tire] -> ActiveTire_FL/2(TMEasy)
  [ASMBUS_VehicleDynamics_ForcesAndTorques_FL_Tire] -> BusCreator1/2
  BusCreator6/1 -> BusCreator3/5  "TireModelSwitch"
  Sw_Tire_Model/1 -> ActiveTire_RR/1(SW_Tire_Model[1TMEasy|2MF]), ActiveTire_RL/1(SW_Tire_Model[1TMEasy|2MF]), ActiveTire_FR/1(SW_Tire_Model[1TMEasy|2MF]), ActiveTire_FL/1(SW_Tire_Model[1TMEasy|2MF]), BusCreator6/1  "Sw_Tire_Model[1TMEasy|2MF]"
  BusCreator5/1 -> BusCreator3/4  "Tire_RR"
  BusCreator4/1 -> BusCreator3/3  "Tire_RL"
  BusCreator2/1 -> BusCreator3/2  "Tire_FR"
  BusCreator1/1 -> BusCreator3/1  "Tire_FL"
  BusCreator3/1 -> ASMSignalBus/1  "Tire"

== system ASM_Traffic_V2X_Complete_Model_2/MDL/VehicleDynamics/Tire/Tire_FL ==
  Coeff_Fric_Road[] : Inport
  " Pos_z_CP_CoorSys_E[m]" : Inport  Port=2
  UnitVec_z_CP_CoorSys_E[x;y;z] : Inport  Port=3
  Pos_Wheels_CoorSys_E[x;y;z][m] : Inport  Port=4
  v_Abs_WheelBody_CoorSys_V[x;y;z][m|s] : Inport  Port=5
  w_Abs_Wheel_CoorSys_V[x;y;z][rad|s] : Inport  Port=6
  RotationMatrix_V_to_E_T[3x3] : Inport  Port=7
  UnitVec_y_Wheel_CoorSys_V[x;y;z] : Inport  Port=8
  omega_Wheel[rad|s] : Inport  Port=9
  Sw_Tire_Parameter_Set[1|2|3|4] : Inport  Port=10
  Sw_Tire_Model[1TMEasy|2MF] : Inport  Port=11
  Reset[] : Inport  Port=12
  Mode[1Normal|2Mirror] : Inport  Port=13
  p[Pa] : Inport  Port=14
  Bus Selector : BusSelector  OutputSignals=Sw_r_Tire[1:intern;2:extern],r_Tire_extern[m]
  CONTACT_POINT_CALCULATION_FL : ASM_VehicleDynamics_lib/VehicleDynamics/Tire/Tire_FL/CONTACT_POINT_CALCULATION_FL  Tag=ASM_SUBCOMPONENT  ASMProperties=struct('Name','CONTACT_POINT_CALCULATION_FL','Version','6.0','Library','ASM_VehicleDynamics_lib')  ASMInstanceName=contact_point_calculation_fl  ASMInstanceID=1
  Demux : Demux  Outputs=[1 1 1 1 1 1 1]
  EnableMF : simulink/Logic and Bit Operations/Compare To Constant  relop=~=  const=2  OutDataTypeStr=boolean  ZeroCross=off
  EnableTMEasy : simulink/Logic and Bit Operations/Compare To Constant  relop===  const=1  OutDataTypeStr=boolean  ZeroCross=off
  IncludedInASMBUS : Terminator
  Multiport Switch : MultiPortSwitch  Inputs=2  SaturateOnIntegerOverflow=on
  Mux : Mux  Inputs=7
  Or : Logic  Operator=OR  AllPortsSameDT=off  OutDataTypeStr=boolean
  TIRE_FORCES_AND_TORQUES_VECTORS_FL : ASM_VehicleDynamics_lib/VehicleDynamics/Tire/Tire_FL/TIRE_FORCES_AND_TORQUES_VECTORS_FL  Tag=ASM_SUBCOMPONENT  ASMProperties=struct('Name','TIRE_FORCES_AND_TORQUES_VECTORS_FL','Version','1.0','Library','ASM_VehicleDynamics_lib')  ASMInstanceName=tire_forces_and_torques_vectors_fl  ASMInstanceID=1
  TIRE_MF : ASM_VehicleDynamics_lib/VehicleDynamics/Tire/TireComponents/TIRE_MF  Tag=ASM_SUBCOMPONENT  Base=MDL.VehicleDynamics.Tire.FL.MF.Base  Para_Set_1=MDL.VehicleDynamics.Tire.FL.MF.Para_Set_1  Para_Set_2=MDL.VehicleDynamics.Tire.FL.MF.Para_Set_2  Para_Set_3=MDL.VehicleDynamics.Tire.FL.MF.Para_Set_3  Para_Set_4=MDL.VehicleDynamics.Tire.FL.MF.Para_Set_4  StepSize=SIM.StepSize  ASMProperties=struct('Name','TIRE_MF','Version','4.0','Library','ASM_VehicleDynamics_lib')  ASMInstanceName=FL  ASMInstanceID=1
      settings: AttributesFormatString=Instance Name: FL\nInstance ID: 1
  TIRE_MODEL_TMEASY_FL : ASM_VehicleDynamics_lib/VehicleDynamics/Tire/Tire_FL/TIRE_MODEL_TMEASY_FL  Tag=ASM_SUBCOMPONENT  Para_Set_1=MDL.VehicleDynamics.Tire.FL.TMEasy.Para_Set_1  Para_Set_2=MDL.VehicleDynamics.Tire.FL.TMEasy.Para_Set_2  Para_Set_3=MDL.VehicleDynamics.Tire.FL.TMEasy.Para_Set_3  Para_Set_4=MDL.VehicleDynamics.Tire.FL.TMEasy.Para_Set_4  StepSize=SIM.StepSize  ASMProperties=struct('Name','TIRE_MODEL_TMEASY_FL','Version','16.0','Library','ASM_VehicleDynamics_lib')  ASMInstanceName=tire_model_tmeasy_fl  ASMInstanceID=1
  F_Tire[x;y;z][N] : Outport
  Trq_Tire[x;y;z][Nm] : Outport  Port=2
  Trq_Tire_Wheel[Nm] : Outport  Port=3
  Stiffness_z_Tire[N|m] : Outport  Port=4
  tag scope: ASMBUS_VehicleDynamics_ContactPoint_FL_Tire=global, ASMBUS_VehicleDynamics_ForcesAndTorques_FL_Tire=global, ASMBUS_VehicleDynamics_MF_FL_Tire=global, ASMBUS_VehicleDynamics_TMEasy_FL_Tire=global
  wires:
  EnableMF/1 -> Or/1
  Or/1 -> TIRE_MF/9
  p[Pa]/1 -> TIRE_MF/13
  Mode[1Normal|2Mirror]/1 -> TIRE_MF/12
  Bus Selector/1 -> TIRE_MODEL_TMEASY_FL/10, TIRE_MF/10  "<Sw_r_Tire[1:intern;2:extern]>"
  Bus Selector/2 -> TIRE_MODEL_TMEASY_FL/11, TIRE_MF/11  "<r_Tire_extern[m]>"
  [TAG_Tire_Switches] -> Bus Selector/1
  Demux/6 -> TIRE_FORCES_AND_TORQUES_VECTORS_FL/6
  Demux/5 -> TIRE_FORCES_AND_TORQUES_VECTORS_FL/5
  Demux/4 -> TIRE_FORCES_AND_TORQUES_VECTORS_FL/4
  Demux/3 -> TIRE_FORCES_AND_TORQUES_VECTORS_FL/3
  Demux/2 -> TIRE_FORCES_AND_TORQUES_VECTORS_FL/2
  Demux/1 -> TIRE_FORCES_AND_TORQUES_VECTORS_FL/1
  Demux/7 -> Stiffness_z_Tire[N|m]/1
  Multiport Switch/1 -> Demux/1
  TIRE_MF/2 -> Multiport Switch/3
  Mux/1 -> Multiport Switch/2
  TIRE_MODEL_TMEASY_FL/8 -> Mux/7
  TIRE_MODEL_TMEASY_FL/7 -> Mux/6
  TIRE_MODEL_TMEASY_FL/6 -> Mux/5
  TIRE_MODEL_TMEASY_FL/5 -> Mux/4
  TIRE_MODEL_TMEASY_FL/4 -> Mux/3
  TIRE_MODEL_TMEASY_FL/3 -> Mux/2
  TIRE_MODEL_TMEASY_FL/2 -> Mux/1
  Reset[]/1 -> CONTACT_POINT_CALCULATION_FL/8, Or/2, TIRE_MODEL_TMEASY_FL/9
  TIRE_FORCES_AND_TORQUES_VECTORS_FL/4 -> Trq_Tire_Wheel[Nm]/1
  TIRE_FORCES_AND_TORQUES_VECTORS_FL/3 -> Trq_Tire[x;y;z][Nm]/1
  TIRE_FORCES_AND_TORQUES_VECTORS_FL/2 -> F_Tire[x;y;z][N]/1
  TIRE_FORCES_AND_TORQUES_VECTORS_FL/1 -> [ASMBUS_VehicleDynamics_ForcesAndTorques_FL_Tire]
  TIRE_MF/1 -> [ASMBUS_VehicleDynamics_MF_FL_Tire]
  TIRE_MODEL_TMEASY_FL/1 -> [ASMBUS_VehicleDynamics_TMEasy_FL_Tire]
  Sw_Tire_Model[1TMEasy|2MF]/1 -> EnableTMEasy/1, EnableMF/1, Multiport Switch/1
  CONTACT_POINT_CALCULATION_FL/1 -> [ASMBUS_VehicleDynamics_ContactPoint_FL_Tire]
  RotationMatrix_V_to_E_T[3x3]/1 -> CONTACT_POINT_CALCULATION_FL/6
  UnitVec_z_CP_CoorSys_E[x;y;z]/1 -> CONTACT_POINT_CALCULATION_FL/5
  " Pos_z_CP_CoorSys_E[m]"/1 -> CONTACT_POINT_CALCULATION_FL/4
  Pos_Wheels_CoorSys_E[x;y;z][m]/1 -> CONTACT_POINT_CALCULATION_FL/3
  w_Abs_Wheel_CoorSys_V[x;y;z][rad|s]/1 -> CONTACT_POINT_CALCULATION_FL/2
  v_Abs_WheelBody_CoorSys_V[x;y;z][m|s]/1 -> CONTACT_POINT_CALCULATION_FL/1
  EnableTMEasy/1 -> TIRE_MODEL_TMEASY_FL/Enable
  CONTACT_POINT_CALCULATION_FL/10 -> TIRE_FORCES_AND_TORQUES_VECTORS_FL/10
  CONTACT_POINT_CALCULATION_FL/9 -> TIRE_FORCES_AND_TORQUES_VECTORS_FL/9
  CONTACT_POINT_CALCULATION_FL/8 -> TIRE_FORCES_AND_TORQUES_VECTORS_FL/8
  CONTACT_POINT_CALCULATION_FL/7 -> TIRE_FORCES_AND_TORQUES_VECTORS_FL/7
  CONTACT_POINT_CALCULATION_FL/11 -> IncludedInASMBUS/1
  CONTACT_POINT_CALCULATION_FL/6 -> TIRE_MODEL_TMEASY_FL/8, TIRE_MF/8
  CONTACT_POINT_CALCULATION_FL/5 -> TIRE_MODEL_TMEASY_FL/7, TIRE_MF/7
  CONTACT_POINT_CALCULATION_FL/4 -> TIRE_MODEL_TMEASY_FL/6, TIRE_MF/6
  CONTACT_POINT_CALCULATION_FL/3 -> TIRE_MODEL_TMEASY_FL/5, TIRE_MF/5
  CONTACT_POINT_CALCULATION_FL/2 -> TIRE_MODEL_TMEASY_FL/4, TIRE_MF/4
  UnitVec_y_Wheel_CoorSys_V[x;y;z]/1 -> TIRE_FORCES_AND_TORQUES_VECTORS_FL/11, CONTACT_POINT_CALCULATION_FL/7
  omega_Wheel[rad|s]/1 -> TIRE_MODEL_TMEASY_FL/3, TIRE_MF/3
  Coeff_Fric_Road[]/1 -> TIRE_MODEL_TMEASY_FL/2, TIRE_MF/2
  Sw_Tire_Parameter_Set[1|2|3|4]/1 -> TIRE_MODEL_TMEASY_FL/1, TIRE_MF/1
